simulink model "eightenPulseRectifier"  (R2024a)
settings: Solver=VariableStepAuto  StartTime=0.0  StopTime=.2  MaxStep=.0001  RelTol=1e-3
libraries: spsThyristorLib x60, spsVoltageMeasurementLib x47, spsControlledVoltageSourceLib x15, spsSeriesRLCBranchLib x9, spsZigzagPhaseShiftingTransformerLib x8, spsGroundLib x6, spsThreePhaseTransformerTwoWindingsLib x4, spsMeanLib x3, spsUniversalBridgeLib x3, slpidlib x1, simulink_extras x1, sps_lib x1
(part 2 of 2)

== system eightenPulseRectifier/Controlled18PulseRectifierLPF_ClosedLoop/Subsystem ==
  freq : Inport
  Vll_RMS : Inport  Port=2
  Add : Sum
  Add1 : Sum
  Add2 : Sum
  Constant : Constant
  Gain : Gain  Gain=2*pi
  Gain1 : Gain  Gain=sqrt(2/3)
  Integrator : Integrator
  Product{,1..3} (4 alike) : Product
  Sin : Trigonometry
  Sin1 : Trigonometry
  Sin2 : Trigonometry
  phase : Constant  Value=0
  phase B : Constant  Value=-2*pi/3
  phase B1 : Constant  Value=2*pi/3
  PhA : Outport
  PhB : Outport  Port=2
  Phc : Outport  Port=3
  wires:
  Sin/1 -> Product/1
  Product3/1 -> Phc/1
  freq/1 -> Product2/1
  Product/1 -> PhA/1
  phase B1/1 -> Add2/2
  Add2/1 -> Sin2/1
  Add1/1 -> Sin1/1
  Add/1 -> Sin/1
  phase B/1 -> Add1/2
  phase/1 -> Add/2
  Vll_RMS/1 -> Gain1/1
  Constant/1 -> Integrator/1
  Integrator/1 -> Gain/1
  Product2/1 -> Add/1, Add1/1, Add2/1
  Product1/1 -> PhB/1
  Sin2/1 -> Product3/1
  Sin1/1 -> Product1/1
  Gain/1 -> Product2/2  "2pit"
  Gain1/1 -> Product1/2, Product3/2, Product/2

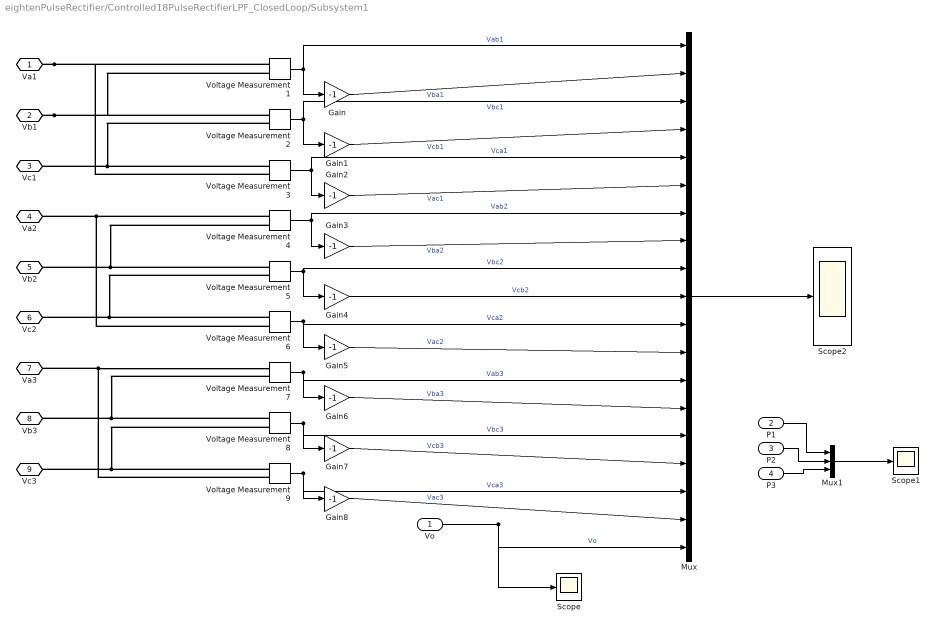
== system eightenPulseRectifier/Controlled18PulseRectifierLPF_ClosedLoop/Subsystem1 ==
  Vo : Inport
  P1 : Inport  Port=2
  P2 : Inport  Port=3
  P3 : Inport  Port=4
  Gain{,1..8} (9 alike) : Gain  Gain=-1
  Mux : Mux  Inputs=19
  Mux1 : Mux  Inputs=3
  Scope : Scope
  Scope1 : Scope
  Scope2 : Scope
  Voltage Measurement{1..9} (9 alike) : spsVoltageMeasurementLib/Voltage Measurement  PhasorSimulation=off  OutputType=Complex  PSBequivalent=0
  Va1 : PMIOPort  Side=Left
  Vb1 : PMIOPort  Port=2  Side=Left
  Vc1 : PMIOPort  Port=3  Side=Left
  Va2 : PMIOPort  Port=4  Side=Left
  Vb2 : PMIOPort  Port=5  Side=Left
  Vc2 : PMIOPort  Port=6  Side=Left
  Va3 : PMIOPort  Port=7  Side=Left
  Vb3 : PMIOPort  Port=8  Side=Left
  Vc3 : PMIOPort  Port=9  Side=Left
  wires:
  Voltage Measurement2/1 -> Gain1/1, Mux/3  "Vbc1"
  Voltage Measurement4/1 -> Gain3/1, Mux/7  "Vab2"
  Voltage Measurement5/1 -> Gain4/1, Mux/9  "Vbc2"
  Voltage Measurement3/1 -> Gain2/1, Mux/5  "Vca1"
  Gain1/1 -> Mux/4  "Vcb1"
  Gain8/1 -> Mux/18  "Vac3"
  Gain7/1 -> Mux/16  "Vcb3"
  Voltage Measurement9/1 -> Mux/17, Gain8/1  "Vca3"
  Gain5/1 -> Mux/12  "Vac2"
  Voltage Measurement7/1 -> Gain6/1, Mux/13  "Vab3"
  Voltage Measurement6/1 -> Gain5/1, Mux/11  "Vca2"
  Voltage Measurement1/1 -> Gain/1, Mux/1  "Vab1"
  Voltage Measurement8/1 -> Mux/15, Gain7/1  "Vbc3"
  Gain4/1 -> Mux/10  "Vcb2"
  Gain2/1 -> Mux/6  "Vac1"
  Gain/1 -> Mux/2  "Vba1"
  Gain6/1 -> Mux/14  "Vba3"
  Gain3/1 -> Mux/8  "Vba2"
  Vo/1 -> Scope/1, Mux/19  "Vo"
  Mux/1 -> Scope2/1
  P1/1 -> Mux1/1
  P2/1 -> Mux1/2
  P3/1 -> Mux1/3
  Mux1/1 -> Scope1/1
  connections:
  Voltage Measurement6/LConn1 -- Voltage Measurement5/LConn2 -- Vc2/RConn1
  Voltage Measurement9/LConn1 -- Voltage Measurement8/LConn2 -- Vc3/RConn1
  Voltage Measurement5/LConn1 -- Voltage Measurement4/LConn2 -- Vb2/RConn1
  Va1/RConn1 -- Voltage Measurement1/LConn1 -- Voltage Measurement3/LConn2
  Voltage Measurement4/LConn1 -- Voltage Measurement6/LConn2 -- Va2/RConn1
  Voltage Measurement9/LConn2 -- Va3/RConn1 -- Voltage Measurement7/LConn1
  Voltage Measurement3/LConn1 -- Voltage Measurement2/LConn2 -- Vc1/RConn1
  Vb1/RConn1 -- Voltage Measurement2/LConn1 -- Voltage Measurement1/LConn2
  Voltage Measurement8/LConn1 -- Voltage Measurement7/LConn2 -- Vb3/RConn1

== system eightenPulseRectifier/Controlled18PulseRectifierLPF_ClosedLoop/Subsystem2 ==
  Three-Phase Transformer (Two Windings) : spsThreePhaseTransformerTwoWindingsLib/Three-Phase Transformer (Two Windings)  Winding1Connection=Yg  Winding2Connection=Yg  CoreType=Three single-phase transformers  SetSaturation=off  Hysteresis=off  DataFile='hysteresis'  SetInitialFlux=off  Measurements=None  UNITS=SI  NominalPower=[ 250e6 , 50 ]  Winding1=[253/sqrt(3) 0 0]  Winding2=[253/sqrt(3) 0 0]  Rm=1.0804e+06  Lm=2866  L0=0.5  Saturation=[0 0;0.66653 1910.3;277.72 2419.7]  InitialFluxes=[ 0.8 , -0.8 , 0.7 ]  BreakLoop=off  DiscreteSolver=Trapezoidal iterative  DataType=on  TransfoNumber=1
  Zigzag Phase-Shifting Transformer : spsZigzagPhaseShiftingTransformerLib/Zigzag Phase-Shifting Transformer  SecondaryConnection=Y  SetSaturation=off  SetInitialFlux=off  Measurements=None  UNITS=SI  NominalPower=[ 100e6 50]  PrimaryVoltage=200/sqrt(3)  SecondaryVoltage="[ 200/sqrt(3)  +20]"  Winding1=[0.000001 0.0000001]  Winding2=[0.000001 0.0000001]  Winding3=[0.000001 0.0000001]  RmLm=[622.01 1.6499]  Rm=622.01  Saturation=[0 0;17.569 28.988;7320.5 36.718]  InitialFluxes=[0 0 0]  BreakLoop=off  DiscreteSolver=Trapezoidal iterative  DataType=on
      settings: LibrarySourceBlock=|
      | sps_lib/Power Grid Elements/Zigzag
      | Phase-Shifting Transformer
  Zigzag Phase-Shifting Transformer1 : spsZigzagPhaseShiftingTransformerLib/Zigzag Phase-Shifting Transformer  SecondaryConnection=Y  SetSaturation=off  SetInitialFlux=off  Measurements=None  UNITS=SI  NominalPower=[ 100e6 50]  PrimaryVoltage=200/sqrt(3)  SecondaryVoltage="[ 200/sqrt(3)  -20]"  Winding1=[0.00001 0.000001]  Winding2=[0.00001 0.000001]  Winding3=[0.00001 0.000001]  RmLm=[622.01 1.6499]  Rm=622.01  Saturation=[0 0;17.569 28.988;7320.5 36.718]  InitialFluxes=[0 0 0]  BreakLoop=off  DiscreteSolver=Trapezoidal iterative  DataType=on
      settings: LibrarySourceBlock=|
      | sps_lib/Power Grid Elements/Zigzag
      | Phase-Shifting Transformer
  A : PMIOPort  Side=Left
  B : PMIOPort  Port=2  Side=Left
  C : PMIOPort  Port=3  Side=Left
  R1 : PMIOPort  Port=4  Side=Right
  S1 : PMIOPort  Port=5  Side=Right
  T1 : PMIOPort  Port=6  Side=Right
  R2 : PMIOPort  Port=7  Side=Right
  S2 : PMIOPort  Port=8  Side=Right
  T2 : PMIOPort  Port=9  Side=Right
  R3 : PMIOPort  Port=10  Side=Right
  S3 : PMIOPort  Port=11  Side=Right
  T3 : PMIOPort  Port=12  Side=Right
  connections:
  Three-Phase Transformer (Two Windings)/LConn3 -- C/RConn1 -- Zigzag Phase-Shifting Transformer/RConn3 -- Zigzag Phase-Shifting Transformer1/RConn3
  Three-Phase Transformer (Two Windings)/RConn1 -- R1/RConn1
  Three-Phase Transformer (Two Windings)/RConn2 -- S1/RConn1
  S2/RConn1 -- Zigzag Phase-Shifting Transformer/LConn2
  Three-Phase Transformer (Two Windings)/LConn2 -- B/RConn1 -- Zigzag Phase-Shifting Transformer/RConn2 -- Zigzag Phase-Shifting Transformer1/RConn2
  T2/RConn1 -- Zigzag Phase-Shifting Transformer/LConn3
  Zigzag Phase-Shifting Transformer1/LConn2 -- S3/RConn1
  Three-Phase Transformer (Two Windings)/RConn3 -- T1/RConn1
  Zigzag Phase-Shifting Transformer1/LConn3 -- T3/RConn1
  Three-Phase Transformer (Two Windings)/LConn1 -- A/RConn1 -- Zigzag Phase-Shifting Transformer/RConn1 -- Zigzag Phase-Shifting Transformer1/RConn1
  Zigzag Phase-Shifting Transformer/LConn6 -- Zigzag Phase-Shifting Transformer/LConn4 -- Zigzag Phase-Shifting Transformer/LConn5
  R2/RConn1 -- Zigzag Phase-Shifting Transformer/LConn1
  Zigzag Phase-Shifting Transformer1/LConn4 -- Zigzag Phase-Shifting Transformer1/LConn6 -- Zigzag Phase-Shifting Transformer1/LConn5
  Zigzag Phase-Shifting Transformer1/LConn1 -- R3/RConn1

== system eightenPulseRectifier/Controlled18PulseRectifierLPF_ClosedLoop/Subsystem3 ==
  P1 : Inport
  Demux : Demux  Outputs=6
  Thyristor{,1..5} (6 alike) : spsThyristorLib/Thyristor  Ron=0.001  Lon=0  Vf=0.8  IC=0  Rs=500  Cs=250e-9  Measurements=off
  + : PMIOPort  Side=Right
  Va : PMIOPort  Port=2  Side=Left
  Vb : PMIOPort  Port=3  Side=Left
  Vc : PMIOPort  Port=4  Side=Left
  - : PMIOPort  Port=5  Side=Right
  wires:
  Demux/1 -> [T1]
  Demux/2 -> [T2]
  Demux/3 -> [T3]
  Demux/4 -> [T4]
  Demux/5 -> [T5]
  Demux/6 -> [T6]
  P1/1 -> Demux/1
  [T1] -> Thyristor/1
  [T3] -> Thyristor1/1
  [T5] -> Thyristor2/1
  [T4] -> Thyristor3/1
  [T2] -> Thyristor5/1
  [T6] -> Thyristor4/1
  connections:
  Thyristor5/RConn1 -- Thyristor2/LConn1 -- Vc/RConn1
  Thyristor3/RConn1 -- Va/RConn1 -- Thyristor/LConn1
  Thyristor/RConn1 -- Thyristor1/RConn1 -- Thyristor2/RConn1 -- +/RConn1
  Thyristor5/LConn1 -- Thyristor4/LConn1 -- Thyristor3/LConn1 -- -/RConn1
  Thyristor4/RConn1 -- Thyristor1/LConn1 -- Vb/RConn1

== system eightenPulseRectifier/Controlled18PulseRectifierLPF_ClosedLoop/Subsystem4 ==
  P1 : Inport
  Demux : Demux  Outputs=6
  Thyristor{,1..5} (6 alike) : spsThyristorLib/Thyristor  Ron=0.001  Lon=0  Vf=0.8  IC=0  Rs=500  Cs=250e-9  Measurements=off
  + : PMIOPort  Side=Right
  Va : PMIOPort  Port=2  Side=Left
  Vb : PMIOPort  Port=3  Side=Left
  Vc : PMIOPort  Port=4  Side=Left
  - : PMIOPort  Port=5  Side=Right
  wires:
  [T6] -> Thyristor4/1
  [T2] -> Thyristor5/1
  [T4] -> Thyristor3/1
  [T5] -> Thyristor2/1
  [T3] -> Thyristor1/1
  [T1] -> Thyristor/1
  P1/1 -> Demux/1
  Demux/6 -> [T6]
  Demux/5 -> [T5]
  Demux/4 -> [T4]
  Demux/3 -> [T3]
  Demux/2 -> [T2]
  Demux/1 -> [T1]
  connections:
  Thyristor1/LConn1 -- Vb/RConn1 -- Thyristor4/RConn1
  -/RConn1 -- Thyristor5/LConn1 -- Thyristor3/LConn1 -- Thyristor4/LConn1
  Thyristor1/RConn1 -- Thyristor/RConn1 -- +/RConn1 -- Thyristor2/RConn1
  Va/RConn1 -- Thyristor/LConn1 -- Thyristor3/RConn1
  Thyristor2/LConn1 -- Vc/RConn1 -- Thyristor5/RConn1

== system eightenPulseRectifier/Controlled18PulseRectifierLPF_ClosedLoop/Subsystem5 ==
  P1 : Inport
  Demux : Demux  Outputs=6
  Thyristor{,1..5} (6 alike) : spsThyristorLib/Thyristor  Ron=0.001  Lon=0  Vf=0.8  IC=0  Rs=500  Cs=250e-9  Measurements=off
  + : PMIOPort  Side=Right
  Va : PMIOPort  Port=2  Side=Left
  Vb : PMIOPort  Port=3  Side=Left
  Vc : PMIOPort  Port=4  Side=Left
  - : PMIOPort  Port=5  Side=Right
  wires:
  Demux/1 -> [T1]
  Demux/2 -> [T2]
  Demux/3 -> [T3]
  Demux/4 -> [T4]
  Demux/5 -> [T5]
  Demux/6 -> [T6]
  P1/1 -> Demux/1
  [T1] -> Thyristor/1
  [T3] -> Thyristor1/1
  [T5] -> Thyristor2/1
  [T4] -> Thyristor3/1
  [T2] -> Thyristor5/1
  [T6] -> Thyristor4/1
  connections:
  Thyristor5/RConn1 -- Vc/RConn1 -- Thyristor2/LConn1
  Thyristor3/RConn1 -- Thyristor/LConn1 -- Va/RConn1
  Thyristor2/RConn1 -- +/RConn1 -- Thyristor/RConn1 -- Thyristor1/RConn1
  Thyristor4/LConn1 -- Thyristor3/LConn1 -- Thyristor5/LConn1 -- -/RConn1
  Thyristor4/RConn1 -- Vb/RConn1 -- Thyristor1/LConn1

== system eightenPulseRectifier/Controlled18PulseRectifierLPF_ClosedLoop/Subsystem6 ==
  delayInDeg : Inport
  Freq : Inport  Port=2
  Add : Sum
  Add1 : Sum  Inputs=+-
  Add2 : Sum
  Constant1 : Constant  Value=360
  Constant4 : Constant  Value=20
  Constant6 : Constant  Value=20
  If : If  IfExpression=u1 < 0
  If Action Subsystem : Subsystem  TreatAsAtomicUnit=on
  If Action Subsystem1 : Subsystem  TreatAsAtomicUnit=on
  Merge : Merge
  Subsystem Reference : Subsystem  ReferencedSubsystem=DoublePulseFor6PulseRectifier
  Subsystem Reference1 : Subsystem  ReferencedSubsystem=DoublePulseFor6PulseRectifier
  Subsystem6 : Subsystem  ReferencedSubsystem=DoublePulseFor6PulseRectifier
  P1 : Outport
  P2 : Outport  Port=2
  P3 : Outport  Port=3
  wires:
  Freq/1 -> Subsystem Reference1/2, Subsystem Reference/2, Subsystem6/2
  Add1/1 -> If Action Subsystem1/1(In1), Add2/1, If/1
  delayInDeg/1 -> Add1/1, Add/1, Subsystem6/1
  Constant4/1 -> Add/2
  Constant6/1 -> Add1/2
  Add/1 -> Subsystem Reference/1
  Subsystem Reference1/1 -> P3/1
  Subsystem6/1 -> P1/1
  Subsystem Reference/1 -> P2/1
  If/1 -> If Action Subsystem/Action
  Add2/1 -> If Action Subsystem/1(In1)
  Constant1/1 -> Add2/2
  If/2 -> If Action Subsystem1/Action
  If Action Subsystem/1(Out1) -> Merge/1
  If Action Subsystem1/1(Out1) -> Merge/2
  Merge/1 -> Subsystem Reference1/1

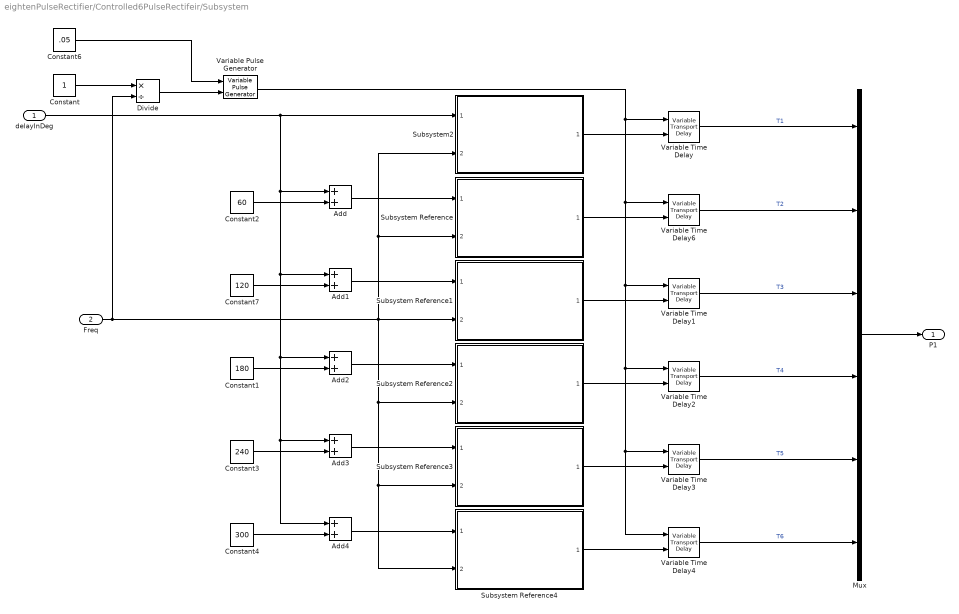
== system eightenPulseRectifier/Controlled6PulseRectifeir/Subsystem ==
  delayInDeg : Inport
  Freq : Inport  Port=2
  Add{,1..4} (5 alike) : Sum
  Constant : Constant
  Constant1 : Constant  Value=180
  Constant2 : Constant  Value=60
  Constant3 : Constant  Value=240
  Constant4 : Constant  Value=300
  Constant6 : Constant  Value=.05
  Constant7 : Constant  Value=120
  Divide : Product  Inputs=*/
  Mux : Mux  Inputs=6
  Subsystem Reference{,1..4} (5 alike) : Subsystem  ReferencedSubsystem=deg2TimeDelay
  Subsystem2 : Subsystem  ReferencedSubsystem=deg2TimeDelay
  Variable Time Delay{,1..4,6} (6 alike) : VariableTransportDelay  MaximumDelay=10  MaximumPoints=20000
  Variable Pulse Generator : VariablePulseGenerator  SampleTime=0.1
  P1 : Outport
  wires:
  Variable Time Delay3/1 -> Mux/5  "T5"
  Variable Pulse Generator/1 -> Variable Time Delay4/1, Variable Time Delay3/1, Variable Time Delay2/1, Variable Time Delay1/1, Variable Time Delay6/1, Variable Time Delay/1
  Freq/1 -> Subsystem2/2, Subsystem Reference/2, Subsystem Reference4/2, Subsystem Reference3/2, Subsystem Reference2/2, Subsystem Reference1/2, Divide/2
  Variable Time Delay6/1 -> Mux/2  "T2"
  Variable Time Delay2/1 -> Mux/4  "T4"
  Variable Time Delay/1 -> Mux/1  "T1"
  Variable Time Delay4/1 -> Mux/6  "T6"
  Subsystem2/1 -> Variable Time Delay/2
  Variable Time Delay1/1 -> Mux/3  "T3"
  Subsystem Reference2/1 -> Variable Time Delay2/2
  Constant2/1 -> Add/2
  Constant1/1 -> Add2/2
  Subsystem Reference1/1 -> Variable Time Delay1/2
  Subsystem Reference4/1 -> Variable Time Delay4/2
  Constant4/1 -> Add4/2
  Subsystem Reference3/1 -> Variable Time Delay3/2
  delayInDeg/1 -> Add4/1, Add3/1, Add2/1, Add1/1, Add/1, Subsystem2/1
  Subsystem Reference/1 -> Variable Time Delay6/2
  Constant3/1 -> Add3/2
  Mux/1 -> P1/1
  Divide/1 -> Variable Pulse Generator/2
  Constant/1 -> Divide/1
  Constant6/1 -> Variable Pulse Generator/1
  Constant7/1 -> Add1/2
  Add1/1 -> Subsystem Reference1/1
  Add/1 -> Subsystem Reference/1
  Add2/1 -> Subsystem Reference2/1
  Add3/1 -> Subsystem Reference3/1
  Add4/1 -> Subsystem Reference4/1

== system eightenPulseRectifier/Controlled6PulseRectifeir/Subsystem4 ==
  P1 : Inport
  Demux : Demux  Outputs=6
  Thyristor{,1..5} (6 alike) : spsThyristorLib/Thyristor  Ron=0.001  Lon=0  Vf=0.8  IC=0  Rs=500  Cs=250e-9  Measurements=off
  + : PMIOPort  Side=Right
  Va : PMIOPort  Port=2  Side=Left
  Vb : PMIOPort  Port=3  Side=Left
  Vc : PMIOPort  Port=4  Side=Left
  - : PMIOPort  Port=5  Side=Right
  wires:
  Demux/1 -> [T1]
  Demux/2 -> [T2]
  Demux/3 -> [T3]
  Demux/4 -> [T4]
  Demux/5 -> [T5]
  Demux/6 -> [T6]
  P1/1 -> Demux/1
  [T1] -> Thyristor/1
  [T3] -> Thyristor1/1
  [T5] -> Thyristor2/1
  [T4] -> Thyristor3/1
  [T2] -> Thyristor5/1
  [T6] -> Thyristor4/1
  connections:
  Thyristor5/RConn1 -- Thyristor2/LConn1 -- Vc/RConn1
  Thyristor3/RConn1 -- Va/RConn1 -- Thyristor/LConn1
  Thyristor/RConn1 -- Thyristor1/RConn1 -- Thyristor2/RConn1 -- +/RConn1
  Thyristor5/LConn1 -- Thyristor4/LConn1 -- Thyristor3/LConn1 -- -/RConn1
  Thyristor4/RConn1 -- Thyristor1/LConn1 -- Vb/RConn1

== system eightenPulseRectifier/Controlled6PulseRectifeir/Subsystem5 ==
  freq : Inport
  Vll_RMS : Inport  Port=2
  Add : Sum
  Add1 : Sum
  Add2 : Sum
  Constant : Constant
  Gain : Gain  Gain=2*pi
  Gain1 : Gain  Gain=sqrt(2/3)
  Integrator : Integrator
  Product{,1..3} (4 alike) : Product
  Sin : Trigonometry
  Sin1 : Trigonometry
  Sin2 : Trigonometry
  phase : Constant  Value=0
  phase B : Constant  Value=-2*pi/3
  phase B1 : Constant  Value=2*pi/3
  PhA : Outport
  PhB : Outport  Port=2
  Phc : Outport  Port=3
  wires:
  Sin/1 -> Product/1
  Product3/1 -> Phc/1
  freq/1 -> Product2/1
  Product/1 -> PhA/1
  phase B1/1 -> Add2/2
  Add2/1 -> Sin2/1
  Add1/1 -> Sin1/1
  Add/1 -> Sin/1
  phase B/1 -> Add1/2
  phase/1 -> Add/2
  Vll_RMS/1 -> Gain1/1
  Constant/1 -> Integrator/1
  Integrator/1 -> Gain/1
  Product2/1 -> Add/1, Add1/1, Add2/1
  Product1/1 -> PhB/1
  Sin2/1 -> Product3/1
  Sin1/1 -> Product1/1
  Gain/1 -> Product2/2  "2pit"
  Gain1/1 -> Product1/2, Product3/2, Product/2

== system eightenPulseRectifier/Uncontrolled18PulseRectifier/Subsystem ==
  freq : Inport
  Vll_RMS : Inport  Port=2
  Add : Sum
  Add1 : Sum
  Add2 : Sum
  Constant : Constant
  Gain : Gain  Gain=2*pi
  Gain1 : Gain  Gain=sqrt(2/3)
  Integrator : Integrator
  Product{,1..3} (4 alike) : Product
  Sin : Trigonometry
  Sin1 : Trigonometry
  Sin2 : Trigonometry
  phase : Constant  Value=0
  phase B : Constant  Value=-2*pi/3
  phase B1 : Constant  Value=2*pi/3
  PhA : Outport
  PhB : Outport  Port=2
  Phc : Outport  Port=3
  wires:
  Gain1/1 -> Product/2, Product3/2, Product1/2
  Gain/1 -> Product2/2  "2pit"
  Sin1/1 -> Product1/1
  Sin2/1 -> Product3/1
  Product1/1 -> PhB/1
  Product2/1 -> Add2/1, Add1/1, Add/1
  Integrator/1 -> Gain/1
  Constant/1 -> Integrator/1
  Vll_RMS/1 -> Gain1/1
  phase/1 -> Add/2
  phase B/1 -> Add1/2
  Add/1 -> Sin/1
  Add1/1 -> Sin1/1
  Add2/1 -> Sin2/1
  phase B1/1 -> Add2/2
  Product/1 -> PhA/1
  freq/1 -> Product2/1
  Product3/1 -> Phc/1
  Sin/1 -> Product/1

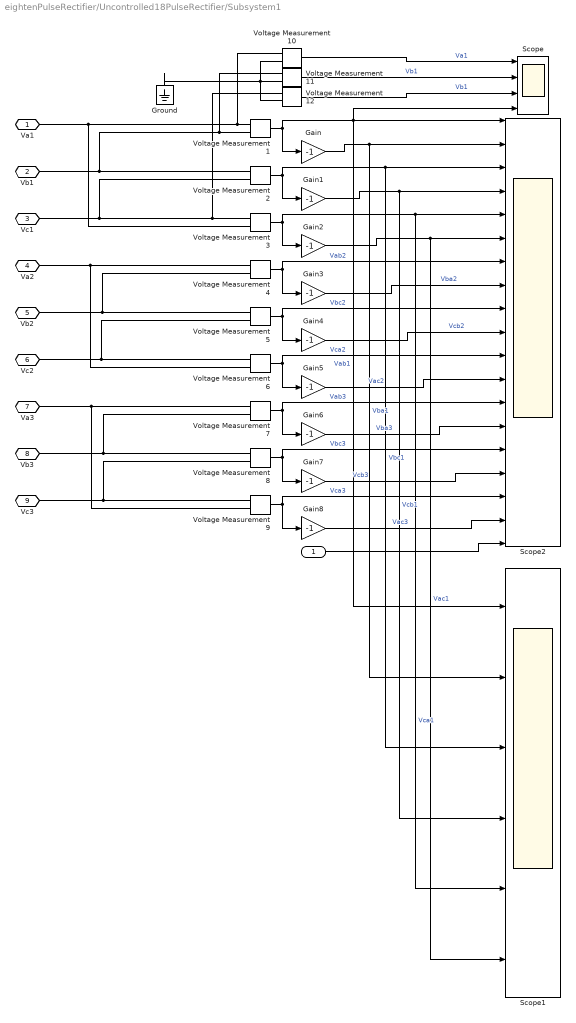
== system eightenPulseRectifier/Uncontrolled18PulseRectifier/Subsystem1 ==
  " " : Inport
  Gain{,1..8} (9 alike) : Gain  Gain=-1
  Ground : spsGroundLib/Ground  LConnTagsString=a
  Scope : Scope  NumInputPorts=4
  Scope1 : Scope  NumInputPorts=6
  Scope2 : Scope  NumInputPorts=19
  Voltage Measurement{1..12} (12 alike) : spsVoltageMeasurementLib/Voltage Measurement  PhasorSimulation=off  OutputType=Complex  PSBequivalent=0
  Va1 : PMIOPort  Side=Left
  Vb1 : PMIOPort  Port=2  Side=Left
  Vc1 : PMIOPort  Port=3  Side=Left
  Va2 : PMIOPort  Port=4  Side=Left
  Vb2 : PMIOPort  Port=5  Side=Left
  Vc2 : PMIOPort  Port=6  Side=Left
  Va3 : PMIOPort  Port=7  Side=Left
  Vb3 : PMIOPort  Port=8  Side=Left
  Vc3 : PMIOPort  Port=9  Side=Left
  wires:
  " "/1 -> Scope2/19
  Voltage Measurement2/1 -> Gain1/1, Scope1/3, Scope2/3  "Vbc1"
  Voltage Measurement4/1 -> Gain3/1, Scope2/7  "Vab2"
  Voltage Measurement5/1 -> Gain4/1, Scope2/9  "Vbc2"
  Voltage Measurement3/1 -> Gain2/1, Scope1/5, Scope2/5  "Vca1"
  Gain1/1 -> Scope1/4, Scope2/4  "Vcb1"
  Gain8/1 -> Scope2/18  "Vac3"
  Gain7/1 -> Scope2/16  "Vcb3"
  Voltage Measurement9/1 -> Gain8/1, Scope2/17  "Vca3"
  Gain5/1 -> Scope2/12  "Vac2"
  Voltage Measurement7/1 -> Gain6/1, Scope2/13  "Vab3"
  Voltage Measurement6/1 -> Gain5/1, Scope2/11  "Vca2"
  Voltage Measurement1/1 -> Gain/1, Scope/4, Scope1/1, Scope2/1  "Vab1"
  Voltage Measurement8/1 -> Gain7/1, Scope2/15  "Vbc3"
  Gain4/1 -> Scope2/10  "Vcb2"
  Gain2/1 -> Scope1/6, Scope2/6  "Vac1"
  Gain/1 -> Scope1/2, Scope2/2  "Vba1"
  Gain6/1 -> Scope2/14  "Vba3"
  Gain3/1 -> Scope2/8  "Vba2"
  Voltage Measurement10/1 -> Scope/1  "Va1"
  Voltage Measurement11/1 -> Scope/2  "Vb1"
  Voltage Measurement12/1 -> Scope/3  "Vb1"
  connections:
  Voltage Measurement6/LConn1 -- Voltage Measurement5/LConn2 -- Vc2/RConn1
  Voltage Measurement8/LConn2 -- Voltage Measurement9/LConn1 -- Vc3/RConn1
  Voltage Measurement5/LConn1 -- Voltage Measurement4/LConn2 -- Vb2/RConn1
  Voltage Measurement1/LConn1 -- Voltage Measurement3/LConn2 -- Va1/RConn1 -- Voltage Measurement10/LConn1
  Voltage Measurement6/LConn2 -- Voltage Measurement4/LConn1 -- Va2/RConn1
  Voltage Measurement9/LConn2 -- Voltage Measurement7/LConn1 -- Va3/RConn1
  Voltage Measurement2/LConn2 -- Voltage Measurement12/LConn1 -- Voltage Measurement3/LConn1 -- Vc1/RConn1
  Voltage Measurement2/LConn1 -- Voltage Measurement1/LConn2 -- Voltage Measurement11/LConn1 -- Vb1/RConn1
  Voltage Measurement7/LConn2 -- Voltage Measurement8/LConn1 -- Vb3/RConn1
  Ground/LConn1 -- Voltage Measurement10/LConn2 -- Voltage Measurement12/LConn2 -- Voltage Measurement11/LConn2

== system eightenPulseRectifier/Uncontrolled18PulseRectifier/Subsystem2 ==
  Three-Phase Transformer (Two Windings) : spsThreePhaseTransformerTwoWindingsLib/Three-Phase Transformer (Two Windings)  Winding1Connection=Yg  Winding2Connection=Yg  CoreType=Three single-phase transformers  SetSaturation=off  Hysteresis=off  DataFile='hysteresis'  SetInitialFlux=off  Measurements=None  UNITS=SI  NominalPower=[ 250e6 , 50 ]  Winding1=[253/sqrt(3) 0 0]  Winding2=[253/sqrt(3) 0 0]  Rm=1.0804e+06  Lm=2866  L0=0.5  Saturation=[0 0;0.66653 1910.3;277.72 2419.7]  InitialFluxes=[ 0.8 , -0.8 , 0.7 ]  BreakLoop=off  DiscreteSolver=Trapezoidal iterative  DataType=on  TransfoNumber=1
  Zigzag Phase-Shifting Transformer : spsZigzagPhaseShiftingTransformerLib/Zigzag Phase-Shifting Transformer  SecondaryConnection=Yg  SetSaturation=off  SetInitialFlux=off  Measurements=None  UNITS=SI  NominalPower=[ 100e6 50]  PrimaryVoltage=200/sqrt(3)  SecondaryVoltage="[ 200/sqrt(3)  +20]"  Winding1=[0.00001 0.000001]  Winding2=[0.00001 0.000001]  Winding3=[0.00001 0.000001]  RmLm=[622.01 1.6499]  Rm=622.01  Saturation=[0 0;17.569 28.988;7320.5 36.718]  InitialFluxes=[0 0 0]  BreakLoop=off  DiscreteSolver=Trapezoidal iterative  DataType=on
      settings: LibrarySourceBlock=|
      | sps_lib/Power Grid Elements/Zigzag
      | Phase-Shifting Transformer
  Zigzag Phase-Shifting Transformer1 : spsZigzagPhaseShiftingTransformerLib/Zigzag Phase-Shifting Transformer  SecondaryConnection=Yg  SetSaturation=off  SetInitialFlux=off  Measurements=None  UNITS=SI  NominalPower=[ 100e6 50]  PrimaryVoltage=200/sqrt(3)  SecondaryVoltage="[ 200/sqrt(3)  -20]"  Winding1=[0.00001 0.000001]  Winding2=[0.00001 0.000001]  Winding3=[0.00001 0.000001]  RmLm=[622.01 1.6499]  Rm=622.01  Saturation=[0 0;17.569 28.988;7320.5 36.718]  InitialFluxes=[0 0 0]  BreakLoop=off  DiscreteSolver=Trapezoidal iterative  DataType=on
      settings: LibrarySourceBlock=|
      | sps_lib/Power Grid Elements/Zigzag
      | Phase-Shifting Transformer
  A : PMIOPort  Side=Left
  B : PMIOPort  Port=2  Side=Left
  C : PMIOPort  Port=3  Side=Left
  R1 : PMIOPort  Port=4  Side=Right
  S1 : PMIOPort  Port=5  Side=Right
  T1 : PMIOPort  Port=6  Side=Right
  R2 : PMIOPort  Port=7  Side=Right
  S2 : PMIOPort  Port=8  Side=Right
  T2 : PMIOPort  Port=9  Side=Right
  R3 : PMIOPort  Port=10  Side=Right
  S3 : PMIOPort  Port=11  Side=Right
  T3 : PMIOPort  Port=12  Side=Right
  connections:
  Zigzag Phase-Shifting Transformer1/RConn3 -- Zigzag Phase-Shifting Transformer/RConn3 -- Three-Phase Transformer (Two Windings)/LConn3 -- C/RConn1
  Three-Phase Transformer (Two Windings)/RConn1 -- R1/RConn1
  Three-Phase Transformer (Two Windings)/RConn2 -- S1/RConn1
  S2/RConn1 -- Zigzag Phase-Shifting Transformer/LConn2
  Three-Phase Transformer (Two Windings)/LConn2 -- B/RConn1 -- Zigzag Phase-Shifting Transformer1/RConn2 -- Zigzag Phase-Shifting Transformer/RConn2
  T2/RConn1 -- Zigzag Phase-Shifting Transformer/LConn3
  Zigzag Phase-Shifting Transformer1/LConn2 -- S3/RConn1
  Three-Phase Transformer (Two Windings)/RConn3 -- T1/RConn1
  Zigzag Phase-Shifting Transformer1/LConn3 -- T3/RConn1
  Three-Phase Transformer (Two Windings)/LConn1 -- A/RConn1 -- Zigzag Phase-Shifting Transformer1/RConn1 -- Zigzag Phase-Shifting Transformer/RConn1
  Zigzag Phase-Shifting Transformer/LConn6 -- Zigzag Phase-Shifting Transformer/LConn4 -- Zigzag Phase-Shifting Transformer/LConn5
  R2/RConn1 -- Zigzag Phase-Shifting Transformer/LConn1
  Zigzag Phase-Shifting Transformer1/LConn6 -- Zigzag Phase-Shifting Transformer1/LConn5 -- Zigzag Phase-Shifting Transformer1/LConn4
  Zigzag Phase-Shifting Transformer1/LConn1 -- R3/RConn1

== system eightenPulseRectifier/Controlled18PulseRectifier/Subsystem6/If Action Subsystem ==
  In1 : Inport
  Action Port : ActionPort  ActionPortLabel=if(u1 < 0)
  Out1 : Outport
  wires:
  In1/1 -> Out1/1

== system eightenPulseRectifier/Controlled18PulseRectifier/Subsystem6/If Action Subsystem1 ==
  In1 : Inport
  Action Port : ActionPort  ActionPortLabel=else
  Out1 : Outport
  wires:
  In1/1 -> Out1/1

== system eightenPulseRectifier/Controlled18PulseRectifierLPF/Subsystem6/If Action Subsystem ==
  In1 : Inport
  Action Port : ActionPort  ActionPortLabel=if(u1 < 0)
  Out1 : Outport
  wires:
  In1/1 -> Out1/1

== system eightenPulseRectifier/Controlled18PulseRectifierLPF/Subsystem6/If Action Subsystem1 ==
  In1 : Inport
  Action Port : ActionPort  ActionPortLabel=else
  Out1 : Outport
  wires:
  In1/1 -> Out1/1

== system eightenPulseRectifier/Controlled18PulseRectifierLPF_ClosedLoop/Subsystem6/If Action Subsystem ==
  In1 : Inport
  Action Port : ActionPort  ActionPortLabel=if(u1 < 0)
  Out1 : Outport
  wires:
  In1/1 -> Out1/1

== system eightenPulseRectifier/Controlled18PulseRectifierLPF_ClosedLoop/Subsystem6/If Action Subsystem1 ==
  In1 : Inport
  Action Port : ActionPort  ActionPortLabel=else
  Out1 : Outport
  wires:
  In1/1 -> Out1/1
